simulink model "MultiPointsTrackingWithPhysicalModel_cs"  (Simulink 8.8)
settings: Solver=ode5  StartTime=0.0  StopTime=40  FixedStep=1/20  RelTol=1e-3
model workspace (MAT data in the model file):
  mbox_table.block_array(1).src = 'built-in/Subsystem'
  mbox_table.block_array(1).dest = 'MultiPointsTrackingWithPhysicalModel_cs/Mazda_RX8_1'
  mbox_table.block_array(1).mode = 0
  mbox_table.block_array(2).src = 'simulink/Sinks/Out1'
  mbox_table.block_array(2).dest = 'MultiPointsTrackingWithPhysicalModel_cs/Mazda_RX8_1/STATE_Mazda_RX8_1'
  mbox_table.block_array(2).mode = 0
  mbox_table.block_array(3).src = 'PreScanSimulinkLibrary/State'
  mbox_table.block_array(3).dest = 'MultiPointsTrackingWithPhysicalModel_cs/STATE_Mazda_RX8_1'
  mbox_table.block_array(3).mode = 0
  mbox_table.block_array(4).src = 'PreScanSimulinkLibrary/SELF'
  mbox_table.block_array(4).dest = 'MultiPointsTrackingWithPhysicalModel_cs/SELF_Mazda_RX8_1'
  mbox_table.block_array(4).mode = 0
  mbox_table.block_array(5).src = 'simulink/Sources/In1'
  mbox_table.block_array(5).dest = 'MultiPointsTrackingWithPhysicalModel_cs/Mazda_RX8_1/SELF_Mazda_RX8_1'
  mbox_table.block_array(5).mode = 0
  mbox_table.block_array(6).src = 'PreScanSimulinkLibrary/DemuxSELF'
  mbox_table.block_array(6).dest = 'MultiPointsTrackingWithPhysicalModel_cs/Mazda_RX8_1/SELF_Demux'
  mbox_table.block_array(6).mode = 0
  mbox_table.block_array(7).src = 'built-in/Subsystem'
  mbox_table.block_array(7).dest = 'MultiPointsTrackingWithPhysicalModel_cs/Mazda_RX8_1/Dynamics_Empty'
  mbox_table.block_array(7).mode = 0
  mbox_table.block_array(8).src = 'PreScanSimulinkLibrary/MuxState'
  mbox_table.block_array(8).dest = 'MultiPointsTrackingWithPhysicalModel_cs/Mazda_RX8_1/Dynamics_Empty/MuxState'
  mbox_table.block_array(8).mode = 0
  mbox_table.block_array(9).src = 'simulink/Sinks/Out1'
  mbox_table.block_array(9).dest = 'MultiPointsTrackingWithPhysicalModel_cs/Mazda_RX8_1/Dynamics_Empty/State'
  mbox_table.block_array(9).mode = 0
  mbox_table.block_array(10).src = 'built-in/Note'
  mbox_table.block_array(10).dest = 'MultiPointsTrackingWithPhysicalModel_cs/Mazda_RX8_1/Dynamics_Empty/For state mode ''Dynamic'' positions
    | are not taken into account, as they
    | are computed by integrating velocity.
    | Click annotation for Help.'
  mbox_table.block_array(10).mode = 0
  mbox_table.block_array(11).src = 'SimCoreLibrary/SimCoreConfiguration'
  mbox_table.block_array(11).dest = 'MultiPointsTrackingWithPhysicalModel_cs/SimCoreConfiguration'
  mbox_table.block_array(11).mode = 0
  mbox_table.block_array(12).src = 'SimCoreLibrary/Actuators'
  mbox_table.block_array(12).dest = 'MultiPointsTrackingWithPhysicalModel_cs/Actuators'
  mbox_table.block_array(12).mode = 0
  mbox_table.block_array(13).src = 'SimCoreLibrary/SetActuators'
  mbox_table.block_array(13).dest = 'MultiPointsTrackingWithPhysicalModel_cs/SetActuators'
  mbox_table.block_array(13).mode = 0
  mbox_table.block_array(14).src = 'SimCoreLibrary/GetSensors'
  mbox_table.block_array(14).dest = 'MultiPointsTrackingWithPhysicalModel_cs/GetSensors'
  mbox_table.block_array(14).mode = 0
  mbox_table.block_array(15).src = 'SimCoreLibrary/SimCoreInfo'
  mbox_table.block_array(15).dest = 'MultiPointsTrackingWithPhysicalModel_cs/SimCoreInfo'
  mbox_table.block_array(15).mode = 0
  mbox_table.block_array(16).src = 'PreScanSimulinkLibrary/Regenerate'
  mbox_table.block_array(16).dest = 'MultiPointsTrackingWithPhysicalModel_cs/Regenerate'
  mbox_table.block_array(16).mode = 0
  mbox_table.block_array(17).src = 'PreScanSimulinkLibrary/Record for Replay  '
  mbox_table.block_array(17).dest = 'MultiPointsTrackingWithPhysicalModel_cs/Record for Replay  '
  mbox_table.block_array(17).mode = 0
  mbox_table.block_array(18).src = 'PreScanSimulinkLibrary/Open Useful Blocks'
  mbox_table.block_array(18).dest = 'MultiPointsTrackingWithPhysicalModel_cs/Open Useful Blocks'
  mbox_table.block_array(18).mode = 0
  mbox_table.block_array(19).src = 'PreScanSimulinkLibrary/PreScan Options   '
  mbox_table.block_array(19).dest = 'MultiPointsTrackingWithPhysicalModel_cs/PreScan Options   '
  mbox_table.block_array(19).mode = 0
  mbox_table.block_array(20).src = 'built-in/Note'
  mbox_table.block_array(20).dest = 'MultiPointsTrackingWithPhysicalModel_cs/Version:                  '
  mbox_table.block_array(20).mode = 0
  mbox_table.block_array(21).src = 'built-in/Note'
  mbox_table.block_array(21).dest = 'MultiPointsTrackingWithPhysicalModel_cs/7.5.1'
  mbox_table.block_array(21).mode = 0
  mbox_table.block_array(22).src = 'built-in/Note'
  mbox_table.block_array(22).dest = 'MultiPointsTrackingWithPhysicalModel_cs/Author(s):                '
  mbox_table.block_array(22).mode = 0
  mbox_table.block_array(23).src = 'built-in/Note'
  mbox_table.block_array(23).dest = 'MultiPointsTrackingWithPhysicalModel_cs/N.A.'
  mbox_table.block_array(23).mode = 0
  mbox_table.block_array(24).src = 'built-in/Note'
  mbox_table.block_array(24).dest = 'MultiPointsTrackingWithPhysicalModel_cs/Descriptive text:      '
  mbox_table.block_array(24).mode = 0
  mbox_table.block_array(25).src = 'built-in/Note'
  mbox_table.block_array(25).dest = 'MultiPointsTrackingWithPhysicalModel_cs/N.A.'
  mbox_table.block_array(25).mode = 0
  mbox_table.block_array(26).src = 'built-in/Note'
  mbox_table.block_array(26).dest = 'MultiPointsTrackingWithPhysicalModel_cs/ID
    | 
    | 1'
  mbox_table.block_array(26).mode = 0
  mbox_table.block_array(27).src = 'built-in/Note'
  mbox_table.block_array(27).dest = 'MultiPointsTrackingWithPhysicalModel_cs/OBU-Beacon ID
    | 
    | '
  mbox_table.block_array(27).mode = 0
  mbox_table.block_array(28).src = 'built-in/Note'
  mbox_table.block_array(28).dest = 'MultiPointsTrackingWithPhysicalModel_cs/TypeID
    | 
    | 1'
  mbox_table.block_array(28).mode = 0
  mbox_table.block_array(29).src = 'built-in/Note'
  mbox_table.block_array(29).dest = 'MultiPointsTrackingWithPhysicalModel_cs/TypeTag
    | 
    | Car'
  mbox_table.block_array(29).mode = 0
  mbox_table.block_array(30).src = 'built-in/Note'
  mbox_table.block_array(30).dest = 'MultiPointsTrackingWithPhysicalModel_cs/SD
    | 
    | Y'
  mbox_table.block_array(30).mode = 0
  mbox_table.block_array(31).src = 'built-in/Note'
  mbox_table.block_array(31).dest = 'MultiPointsTrackingWithPhysicalModel_cs/CD
    | 
    | N'
  mbox_table.block_array(31).mode = 0
  mbox_table.block_array(32).src = 'built-in/Note'
  mbox_table.block_array(32).dest = 'MultiPointsTrackingWithPhysicalModel_cs/Name
    | 
    | Mazda_RX8_1'
  mbox_table.block_array(32).mode = 0
  mbox_table.block_array(33).src = 'built-in/Note'
  mbox_table.block_array(33).dest = 'MultiPointsTrackingWithPhysicalModel_cs/Num ID       OBU-Beacon ID     Type ID      Type Tag             SD        CD             Name                          '
  mbox_table.block_array(33).mode = 0
  mbox_table.block_array(34).src = 'built-in/Ground'
  mbox_table.block_array(34).dest = 'MultiPointsTrackingWithPhysicalModel_cs/Mazda_RX8_1/Dynamics_Empty/Ground_1'
  mbox_table.block_array(34).mode = 1
  mbox_table.block_array(35).src = 'built-in/Ground'
  mbox_table.block_array(35).dest = 'MultiPointsTrackingWithPhysicalModel_cs/Mazda_RX8_1/Dynamics_Empty/Ground_2'
  mbox_table.block_array(35).mode = 1
  mbox_table.block_array(36).src = 'built-in/Ground'
  mbox_table.block_array(36).dest = 'MultiPointsTrackingWithPhysicalModel_cs/Mazda_RX8_1/Dynamics_Empty/Ground_3'
  mbox_table.block_array(36).mode = 1
  mbox_table.block_array(37).src = 'built-in/Ground'
  mbox_table.block_array(37).dest = 'MultiPointsTrackingWithPhysicalModel_cs/Mazda_RX8_1/Dynamics_Empty/Ground_4'
  mbox_table.block_array(37).mode = 1
  mbox_table.block_array(38).src = 'built-in/Terminator'
  mbox_table.block_array(38).dest = 'MultiPointsTrackingWithPhysicalModel_cs/Mazda_RX8_1/Terminator_1'
  mbox_table.block_array(38).mode = 1
  mbox_table.block_array(39).src = 'built-in/Terminator'
  mbox_table.block_array(39).dest = 'MultiPointsTrackingWithPhysicalModel_cs/Mazda_RX8_1/Terminator_2'
  mbox_table.block_array(39).mode = 1
  mbox_table.block_array(40).src = 'built-in/Terminator'
  mbox_table.block_array(40).dest = 'MultiPointsTrackingWithPhysicalModel_cs/Mazda_RX8_1/Terminator_3'
  mbox_table.block_array(40).mode = 1
  mbox_table.block_array(41).src = 'built-in/Terminator'
  mbox_table.block_array(41).dest = 'MultiPointsTrackingWithPhysicalModel_cs/Mazda_RX8_1/Terminator_4'
  mbox_table.block_array(41).mode = 1
  mbox_table.block_array(42).src = 'built-in/Terminator'
  mbox_table.block_array(42).dest = 'MultiPointsTrackingWithPhysicalModel_cs/Mazda_RX8_1/Terminator_5'
  mbox_table.block_array(42).mode = 1
  mbox_table.block_array(43).src = 'built-in/Terminator'
  mbox_table.block_array(43).dest = 'MultiPointsTrackingWithPhysicalModel_cs/Mazda_RX8_1/Terminator_6'
  mbox_table.block_array(43).mode = 1
  mbox_table.block_array(44).src = 'built-in/Terminator'
  mbox_table.block_array(44).dest = 'MultiPointsTrackingWithPhysicalModel_cs/Mazda_RX8_1/Terminator_7'
  mbox_table.block_array(44).mode = 1
  mbox_table.block_array(45).src = 'built-in/Terminator'
  mbox_table.block_array(45).dest = 'MultiPointsTrackingWithPhysicalModel_cs/Mazda_RX8_1/Terminator_8'
  mbox_table.block_array(45).mode = 1
  mbox_table.block_index : java.util.Hashtable (value not decoded)
  mbox_table.line_array(1).sys = 'MultiPointsTrackingWithPhysicalModel_cs'
  mbox_table.line_array(1).line_id = 'L1'
  mbox_table.line_array(1).iport = 'STATE_Mazda_RX8_1/1'
  mbox_table.line_array(1).oport = 'Mazda_RX8_1/1'
  mbox_table.line_array(1).mode = 0
  mbox_table.line_array(2).sys = 'MultiPointsTrackingWithPhysicalModel_cs'
  mbox_table.line_array(2).line_id = 'L2'
  mbox_table.line_array(2).iport = 'Mazda_RX8_1/1'
  mbox_table.line_array(2).oport = 'SELF_Mazda_RX8_1/1'
  mbox_table.line_array(2).mode = 0
  mbox_table.line_array(3).sys = 'MultiPointsTrackingWithPhysicalModel_cs/Mazda_RX8_1'
  mbox_table.line_array(3).line_id = 'L3'
  mbox_table.line_array(3).iport = 'SELF_Demux/1'
  mbox_table.line_array(3).oport = 'SELF_Mazda_RX8_1/1'
  mbox_table.line_array(3).mode = 0
  mbox_table.line_array(4).sys = 'MultiPointsTrackingWithPhysicalModel_cs/Mazda_RX8_1/Dynamics_Empty'
  mbox_table.line_array(4).line_id = 'L4'
  mbox_table.line_array(4).iport = 'State/1'
  mbox_table.line_array(4).oport = 'MuxState/1'
  mbox_table.line_array(4).mode = 0
  mbox_table.line_array(5).sys = 'MultiPointsTrackingWithPhysicalModel_cs/Mazda_RX8_1'
  mbox_table.line_array(5).line_id = 'L5'
  mbox_table.line_array(5).iport = 'STATE_Mazda_RX8_1/1'
  mbox_table.line_array(5).oport = 'Dynamics_Empty/1'
  mbox_table.line_array(5).mode = 0
  mbox_table.line_array(6).sys = 'MultiPointsTrackingWithPhysicalModel_cs/Mazda_RX8_1/Dynamics_Empty'
  mbox_table.line_array(6).line_id = 'l1'
  mbox_table.line_array(6).iport = 'MuxState/3'
  mbox_table.line_array(6).oport = 'Ground_1/1'
  mbox_table.line_array(6).mode = 1
  mbox_table.line_array(7).sys = 'MultiPointsTrackingWithPhysicalModel_cs/Mazda_RX8_1/Dynamics_Empty'
  mbox_table.line_array(7).line_id = 'l2'
  mbox_table.line_array(7).iport = 'MuxState/6'
  mbox_table.line_array(7).oport = 'Ground_2/1'
  mbox_table.line_array(7).mode = 1
  mbox_table.line_array(8).sys = 'MultiPointsTrackingWithPhysicalModel_cs/Mazda_RX8_1/Dynamics_Empty'
  mbox_table.line_array(8).line_id = 'l3'
  mbox_table.line_array(8).iport = 'MuxState/7'
  mbox_table.line_array(8).oport = 'Ground_3/1'
  mbox_table.line_array(8).mode = 1
  mbox_table.line_array(9).sys = 'MultiPointsTrackingWithPhysicalModel_cs/Mazda_RX8_1/Dynamics_Empty'
  mbox_table.line_array(9).line_id = 'l4'
  mbox_table.line_array(9).iport = 'MuxState/8'
  mbox_table.line_array(9).oport = 'Ground_4/1'
  mbox_table.line_array(9).mode = 1
  mbox_table.line_array(10).sys = 'MultiPointsTrackingWithPhysicalModel_cs/Mazda_RX8_1'
  mbox_table.line_array(10).line_id = 'l5'
  mbox_table.line_array(10).iport = 'Terminator_1/1'
  mbox_table.line_array(10).oport = 'SELF_Demux/3'
  mbox_table.line_array(10).mode = 1
  mbox_table.line_array(11).sys = 'MultiPointsTrackingWithPhysicalModel_cs/Mazda_RX8_1'
  mbox_table.line_array(11).line_id = 'l6'
  mbox_table.line_array(11).iport = 'Terminator_2/1'
  mbox_table.line_array(11).oport = 'SELF_Demux/4'
  mbox_table.line_array(11).mode = 1
  mbox_table.line_array(12).sys = 'MultiPointsTrackingWithPhysicalModel_cs/Mazda_RX8_1'
  mbox_table.line_array(12).line_id = 'l7'
  mbox_table.line_array(12).iport = 'Terminator_3/1'
  mbox_table.line_array(12).oport = 'SELF_Demux/5'
  mbox_table.line_array(12).mode = 1
  mbox_table.line_array(13).sys = 'MultiPointsTrackingWithPhysicalModel_cs/Mazda_RX8_1'
  mbox_table.line_array(13).line_id = 'l8'
  mbox_table.line_array(13).iport = 'Terminator_4/1'
  mbox_table.line_array(13).oport = 'SELF_Demux/7'
  mbox_table.line_array(13).mode = 1
  mbox_table.line_array(14).sys = 'MultiPointsTrackingWithPhysicalModel_cs/Mazda_RX8_1'
  mbox_table.line_array(14).line_id = 'l9'
  mbox_table.line_array(14).iport = 'Terminator_5/1'
  mbox_table.line_array(14).oport = 'SELF_Demux/8'
  mbox_table.line_array(14).mode = 1
  mbox_table.line_array(15).sys = 'MultiPointsTrackingWithPhysicalModel_cs/Mazda_RX8_1'
  mbox_table.line_array(15).line_id = 'l10'
  mbox_table.line_array(15).iport = 'Terminator_6/1'
  mbox_table.line_array(15).oport = 'SELF_Demux/9'
  mbox_table.line_array(15).mode = 1
  mbox_table.line_array(16).sys = 'MultiPointsTrackingWithPhysicalModel_cs/Mazda_RX8_1'
  mbox_table.line_array(16).line_id = 'l11'
  mbox_table.line_array(16).iport = 'Terminator_7/1'
  mbox_table.line_array(16).oport = 'SELF_Demux/10'
  mbox_table.line_array(16).mode = 1
  mbox_table.line_array(17).sys = 'MultiPointsTrackingWithPhysicalModel_cs/Mazda_RX8_1'
  mbox_table.line_array(17).line_id = 'l12'
  mbox_table.line_array(17).iport = 'Terminator_8/1'
  mbox_table.line_array(17).oport = 'SELF_Demux/12'
  mbox_table.line_array(17).mode = 1
  mbox_table.line_index : java.util.Hashtable (value not decoded)
  mbox_table.next_linenr = 6
  mbox_table.next_termlinenr = 13
  model_closed = 0
  sim_status = 0
PreLoadFcn:
  | check_NUTS_defined;
  | 
  | assignin('base',['model_closed_' bdroot],false);
InitFcn:
  | PreScanExperimentInitFcn(bdroot)
StopFcn:
  | PreScanExperimentStopFcn(bdroot)
undefined symbols (not defined in the file): DiscIntNeverNeededParam, lf, lr
libraries: PreScanSimulinkLibrary x2, PreScanUsefulBlocks x1
CloseFcn:
  | evalin('base',['clear model_closed_' bdroot]);
settings Model: Creator=PRESCAN  LastModifiedBy=yuntao891011
settings OptimizationCC: ExpressionDepthLimit=2147483647  InitFltsAndDblsToZero=on
settings DebuggingCC: SaveWithParameterizedLinksMsg=none  SignalResolutionControl=TryResolveAllWithWarning  MultiTaskDSMMsg=warning  MultiTaskCondExecSysMsg=none
settings GRTTargetCC: TargetFcnLib=ansi_tfl_tmw.mat

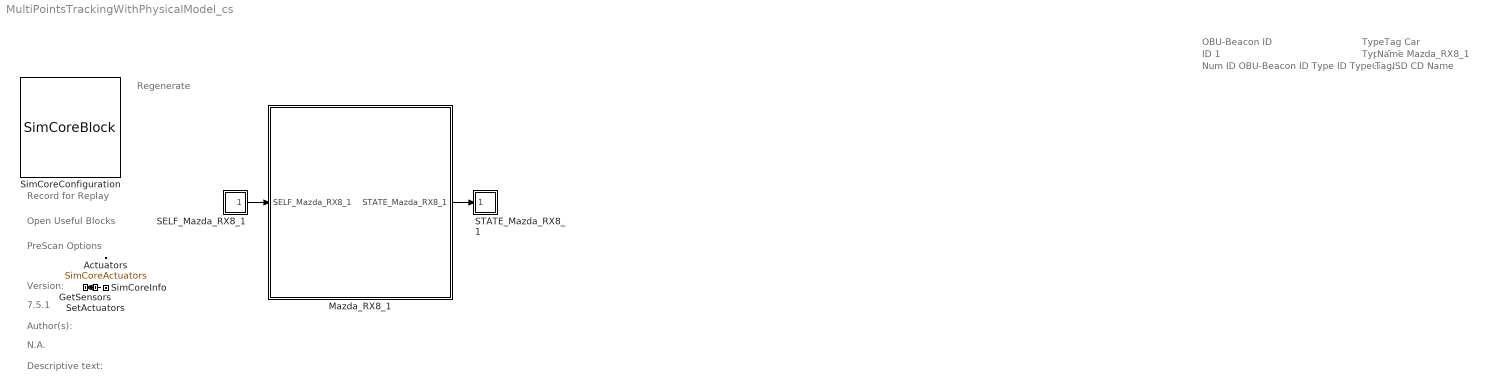
== system MultiPointsTrackingWithPhysicalModel_cs ==
  note: Regenerate
  note: Record for Replay
  note: Open Useful Blocks
  note: PreScan Options
  note: Version:
  note: 7.5.1
  note: Author(s):
  note: N.A.
  note: Descriptive text:
  note: ID
      |
      | 1
  note: OBU-Beacon ID
  note: TypeID
      |
      | 1
  note: TypeTag
      |
      | Car
  note: SD
      |
      | Y
  note: CD
      |
      | N
  note: Name
      |
      | Mazda_RX8_1
  note: Num ID OBU-Beacon ID Type ID Type Tag SD CD Name
  Actuators : DataStoreMemory  DataStoreName=SimCoreActuators  InitialValue=zeros(15,1)  ShowAdditionalParam=off
  GetSensors : Subsystem  Tag=GetSensors  Priority=2  mask(PreScan Simulation Core Block){NrOfSensors=8, TimeStep=1/20}
      mask prompts: NrOfSensors "Number of sensor values"; TimeStep "Timestep [s]"
      mask help:
      | Please do not remove this block from the PreScan compilation sheet,
      | as it contains essential configuration parameters for a PreScan simulation.
      settings: DeleteFcn=PreScanBlockDeleteFcn;
  Mazda_RX8_1 : Subsystem  Tag=WorldObjectSubSystem  InitFcn=UniqueId = '13';
      mask Display: image(imread('Mazda_RX8.jpg'));color('white');text(0,0,' ID=1\n')
  SELF_Mazda_RX8_1 : Subsystem  Tag=SELF  Priority=3  mask(PreScan Source Block: SELF){PortName=SELF_Mazda_RX8_1, PortIndex=0, PortWidth=8, TimeStep=1/20}
      mask prompts: PortName "Auto-Assigned: Port Name [-]"; PortIndex "Auto-Assigned: Port Index [-]"; PortWidth "Auto-Assigned: Port Dimensions"; TimeStep "Auto-Assigned: Upload Period [s]"
      mask help:
      | The SELF port shows (state) information of the actor itself. The outputs are position in the experiment's axis system and the GPS coordinates, and the object's absolute velocity and compass heading.
      |
      | For more information, please click Help.
      settings: DeleteFcn=PreScanBlockDeleteFcn;
      mask Help: eval('openHelp(462)')
      mask Display: image(imread('GPS.png'))
  STATE_Mazda_RX8_1 : Subsystem  Tag=State  Priority=0  mask(PreScan Sink Block: State){x0=34.980075836181641, y0=20.47808837890625, z0=0.51, Roll0=0, Pitch0=0, Yaw0=0, TimeStep=1/20}
      mask prompts: x0 "Ini x-position VEHICLE wrt GLOBAL axis system [m]"; y0 "Ini y-position VEHICLE wrt GLOBAL axis system [m]"; z0 "Ini z-position VEHICLE wrt GLOBAL axis system [m]"; Roll0 "Ini roll-angle BODY wrt VEHICLE axis system [deg]"; Pitch0 "Ini pitch-angle BODY wrt VEHICLE axis system [deg]"; Yaw0 "Ini yaw-angle VEHICLE wrt GLOBAL axis system [deg]"; TimeStep "Time Step [s]"
      mask help:
      | The Actor State contains a vector signal of size (9x1), containing the following signals:
      |
      | -  Position                  (x,y,z)                                     [m]
      | -  Velocity                  (vx,vy,vz)                               [m/s]
      | -  Angles                    (Roll, Pitch, Yaw)                   [rad]
      |
      | The Actor state is defined in the global axis system.
      | The state is superponed on the Initial position defined in the GUI.
      |
      | For more information, please click Help.
      settings: DeleteFcn=PreScanBlockDeleteFcn;
      mask Help: eval('openHelp(222)')
      mask Display: image(imread('State.png'))
  SetActuators : Subsystem  Tag=SetActuators  Priority=1  mask(PreScan Simulation Core Block){TimeStep=1/20, NrOfActuators=15}
      mask prompts: TimeStep "Timestep [s]"; NrOfActuators "Number of actuator values"
      mask help:
      | Please do not remove this block from the PreScan compilation sheet,
      | as it contains essential configuration parameters for a PreScan simulation.
      settings: DeleteFcn=PreScanBlockDeleteFcn;
  SimCoreConfiguration : M-S-Function  Tag=SimCoreConfiguration  Description=C94D2F6BE556C758A06BE63D65435D148AE299C2DC3E9AB8226DE295F427155E  FunctionName=SimCoreBlock  Parameters=ExperimentXML PortsXML SimulationCore HostName CheckStart EnableLog RfR EnableGPUAccel ShowComputationTime  mask(PreScan Simulation Core Configurator){SimulationCore=NUTS, HostName=0, CheckStart=0, prescanversion='7.5.1', EnableLog=off, RfR=0, EnableGPUAccel=off, ShowComputationTime=off}
      mask prompts: SimulationCore "Simulation Core"; HostName "Simulation Host"; CheckStart "Show START Dialog"; prescanversion "PreScan Version"; EnableLog "Create TA Log"; RfR "Record for Replay"; EnableGPUAccel "Enable GPU Acceleration"; ShowComputationTime "Show ComputationTime Scope"
      mask help:
      | Please do not remove this block from the PreScan compilation sheet,
      | as it contains essential configuration parameter for a PreScan simulation.
      mask init:
      | model = bdroot;
      | ExperimentXML = [model(1:end-3) '.pex'];
      | PortsXML = [model '_ports.pcd'];
      settings: DeleteFcn=PreScanBlockDeleteFcn;  ModelCloseFcn=assignin('base',['model_closed_' bdroot],true);
      mask Help: eval('openHelp(812)')
      mask Display: image(imread('prescanlogo.ico'))
  SimCoreInfo : Subsystem  Tag=SimCoreInfo
  wires:
  SetActuators/1(dummy) -> GetSensors/1(dummy)
  Mazda_RX8_1/1(STATE_Mazda_RX8_1) -> STATE_Mazda_RX8_1/1(State)
  SELF_Mazda_RX8_1/1(U) -> Mazda_RX8_1/1(SELF_Mazda_RX8_1)

== system MultiPointsTrackingWithPhysicalModel_cs/GetSensors ==
  dummy : Inport
  GetSensors : M-S-Function  FunctionName=GetSensorsBlock  Parameters=TimeStep NrOfSensors
  tag scope: SimCoreSensors=global
  wires:
  GetSensors/1 -> [SimCoreSensors]
  dummy/1 -> GetSensors/1

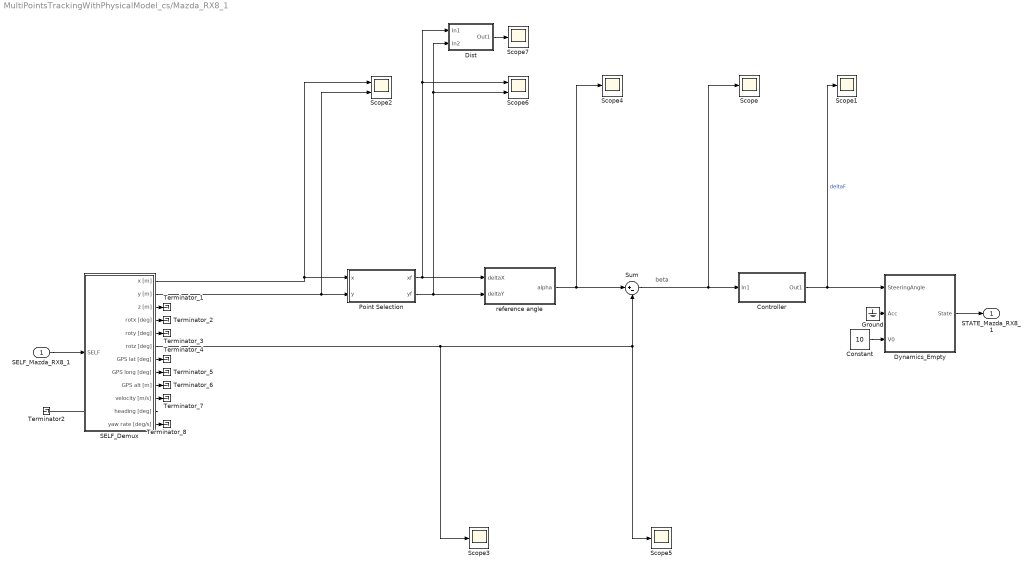
== system MultiPointsTrackingWithPhysicalModel_cs/Mazda_RX8_1 ==
  note: beta
  SELF_Mazda_RX8_1 : Inport  Tag=SELFInport
  Constant : Constant  Value=10
  Controller : Subsystem
  Dist : Subsystem
  Dynamics_Empty : Subsystem  Tag=Dynamics_Empty
      mask Display: port_label('output', 1, 'State');text(0,0,' Empty\n')
  Ground : Ground
  Point Selection : Subsystem
  SELF_Demux : Subsystem  Tag=DemuxSELF  mask(PreScan Demux Block:){}
      settings: DeleteFcn=PreScanBlockDeleteFcn;
      mask Display:
      | port_label('output',1,'x [m]')
      | port_label('output',2,'y [m]')
      | port_label('output',3,'z [m]','texmode','on')
      | port_label('output',4,'Rotx [deg]','texmode','on')
      | port_label('output',5,'Roty [deg]','texmode','on')
      | port_label('output',6,'Rotz [deg]','texmode','on')
      | port_label('output',7,'GPS lat [deg]','texmode','on')
      | port_label('output',8,'GPS long [deg]','texmode','on')
      | port_label('output',9,'GPS alt [m]','texmode','on')
      | port_label('output',10,'Velocity [m/s]')
      | port_label('output',11,'Heading [deg]')
      | port_label('output',12,'Yaw rate [deg/s]')
  Scope{,1,3..5,7} (6 alike) : Scope
  Scope2 : Scope  NumInputPorts=2
  Scope6 : Scope  NumInputPorts=2
  Sum : Sum  Inputs=|+-
  Terminator2 : Terminator
  Terminator_{1..8} (8 alike) : Terminator
  reference angle : Subsystem
  STATE_Mazda_RX8_1 : Outport  Tag=StateOutport
  wires:
  SELF_Demux/1(x [m]) -> Scope2/1, Point Selection/1(x)
  SELF_Demux/2(y [m]) -> Point Selection/2(y), Scope2/2
  Constant/1 -> Dynamics_Empty/3(V0)
  Ground/1 -> Dynamics_Empty/2("Acc ")
  reference angle/1(alpha) -> Sum/1, Scope4/1
  Sum/1 -> Controller/1(In1), Scope/1
  Controller/1(Out1) -> Dynamics_Empty/1(SteeringAngle), Scope1/1  "deltaF"
  SELF_Demux/6(rotz [deg]) -> Scope5/1, Sum/2, Scope3/1
  SELF_Demux/11(heading [deg]) -> Terminator2/1
  Point Selection/1(xf) -> reference angle/1(deltaX), Dist/1(In1), Scope6/1
  Point Selection/2(yf) -> reference angle/2(deltaY), Dist/2(In2), Scope6/2
  Dist/1(Out1) -> Scope7/1
  SELF_Mazda_RX8_1/1 -> SELF_Demux/1(SELF)
  Dynamics_Empty/1(State) -> STATE_Mazda_RX8_1/1
  SELF_Demux/3(z [m]) -> Terminator_1/1
  SELF_Demux/4(rotx [deg]) -> Terminator_2/1
  SELF_Demux/5(roty [deg]) -> Terminator_3/1
  SELF_Demux/7(GPS lat [deg]) -> Terminator_4/1
  SELF_Demux/8(GPS long [deg]) -> Terminator_5/1
  SELF_Demux/9(GPS alt [m]) -> Terminator_6/1
  SELF_Demux/10(velocity [m/s]) -> Terminator_7/1
  SELF_Demux/12(yaw rate [deg/s]) -> Terminator_8/1

== system MultiPointsTrackingWithPhysicalModel_cs/SELF_Mazda_RX8_1 ==
  Selector : Selector  IndexMode=Zero-based  IndexOptions=Starting index (dialog)  Indices=PortIndex  OutputSizes=PortWidth(1)
  U : Outport
  wires:
  Selector/1 -> U/1
  [SimCoreSensors] -> Selector/1

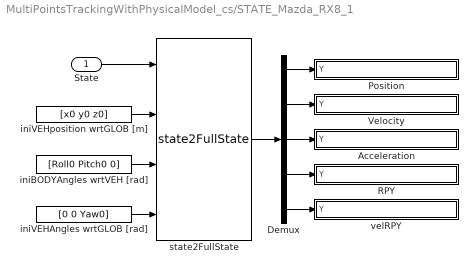
== system MultiPointsTrackingWithPhysicalModel_cs/STATE_Mazda_RX8_1 ==
  State : Inport  SampleTime=TimeStep
  Acceleration : Subsystem  mask(ToSensorWorld){PortName=Acceleration_Mazda_RX8_1, PortIndex=6, PortWidth=3, TimeStep=1/20}
      mask prompts: PortName "Port Name [-]"; PortIndex "Index [-]"; PortWidth "Port Dimensions [-]"; TimeStep "Upload Period [s]"
      mask help: Sends signal(s) from Simulink to the Sensor World
      mask Help:
      | Sends signal(s) from Simulink to the Sensor World.
      | 
      | - Port Name [-]: specifies the name of the output terminal of the Simulink block.
      | - Index [-]: specifies the start position in the output vector sent to the Sensor World
      | - Port dimensions [-]: specifies the width (number of scalars) of the output port
      | - Upload period [s]: specifies the upload period (in seconds) of the port.
      mask Display: port_label('input', 1, PortName)
  Demux : Demux  Outputs=5
  Position : Subsystem  mask(ToSensorWorld){PortName=Position_Mazda_RX8_1, PortIndex=0, PortWidth=3, TimeStep=1/20}
      mask prompts: PortName "Port Name [-]"; PortIndex "Index [-]"; PortWidth "Port Dimensions [-]"; TimeStep "Upload Period [s]"
      mask help: Sends signal(s) from Simulink to the Sensor World
      mask Help:
      | Sends signal(s) from Simulink to the Sensor World.
      | 
      | - Port Name [-]: specifies the name of the output terminal of the Simulink block.
      | - Index [-]: specifies the start position in the output vector sent to the Sensor World
      | - Port dimensions [-]: specifies the width (number of scalars) of the output port
      | - Upload period [s]: specifies the upload period (in seconds) of the port.
      mask Display: port_label('input', 1, PortName)
  RPY : Subsystem  mask(ToSensorWorld){PortName=RPY_Mazda_RX8_1, PortIndex=9, PortWidth=3, TimeStep=1/20}
      mask prompts: PortName "Port Name [-]"; PortIndex "Index [-]"; PortWidth "Port Dimensions [-]"; TimeStep "Upload Period [s]"
      mask help: Sends signal(s) from Simulink to the Sensor World
      mask Help:
      | Sends signal(s) from Simulink to the Sensor World.
      | 
      | - Port Name [-]: specifies the name of the output terminal of the Simulink block.
      | - Index [-]: specifies the start position in the output vector sent to the Sensor World
      | - Port dimensions [-]: specifies the width (number of scalars) of the output port
      | - Upload period [s]: specifies the upload period (in seconds) of the port.
      mask Display: port_label('input', 1, PortName)
  Velocity : Subsystem  mask(ToSensorWorld){PortName=Velocity_Mazda_RX8_1, PortIndex=3, PortWidth=3, TimeStep=1/20}
      mask prompts: PortName "Port Name [-]"; PortIndex "Index [-]"; PortWidth "Port Dimensions [-]"; TimeStep "Upload Period [s]"
      mask help: Sends signal(s) from Simulink to the Sensor World
      mask Help:
      | Sends signal(s) from Simulink to the Sensor World.
      | 
      | - Port Name [-]: specifies the name of the output terminal of the Simulink block.
      | - Index [-]: specifies the start position in the output vector sent to the Sensor World
      | - Port dimensions [-]: specifies the width (number of scalars) of the output port
      | - Upload period [s]: specifies the upload period (in seconds) of the port.
      mask Display: port_label('input', 1, PortName)
  iniBODYAngles wrtVEH [rad] : Constant  Value=[Roll0 Pitch0 0]  SampleTime=TimeStep
  iniVEHAngles wrtGLOB [rad] : Constant  Value=[0 0 Yaw0]  SampleTime=TimeStep
  iniVEHposition wrtGLOB [m] : Constant  Value=[x0 y0 z0]  SampleTime=TimeStep
  state2FullState : PreScanSimulinkLibrary/state2FullState  SystemSampleTime=-1
  velRPY : Subsystem  mask(ToSensorWorld){PortName=velRPY_Mazda_RX8_1, PortIndex=12, PortWidth=3, TimeStep=1/20}
      mask prompts: PortName "Port Name [-]"; PortIndex "Index [-]"; PortWidth "Port Dimensions [-]"; TimeStep "Upload Period [s]"
      mask help: Sends signal(s) from Simulink to the Sensor World
      mask Help:
      | Sends signal(s) from Simulink to the Sensor World.
      | 
      | - Port Name [-]: specifies the name of the output terminal of the Simulink block.
      | - Index [-]: specifies the start position in the output vector sent to the Sensor World
      | - Port dimensions [-]: specifies the width (number of scalars) of the output port
      | - Upload period [s]: specifies the upload period (in seconds) of the port.
      mask Display: port_label('input', 1, PortName)
  wires:
  Demux/5 -> velRPY/1(Y)
  Demux/4 -> RPY/1(Y)
  Demux/3 -> Acceleration/1(Y)
  Demux/2 -> Velocity/1(Y)
  Demux/1 -> Position/1(Y)
  State/1 -> state2FullState/1
  state2FullState/1 -> Demux/1
  iniVEHposition wrtGLOB [m]/1 -> state2FullState/2
  iniBODYAngles wrtVEH [rad]/1 -> state2FullState/3
  iniVEHAngles wrtGLOB [rad]/1 -> state2FullState/4

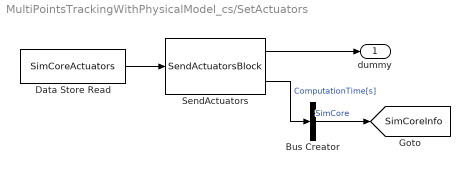
== system MultiPointsTrackingWithPhysicalModel_cs/SetActuators ==
  Bus Creator : BusCreator  Inputs=1
  Data Store Read : DataStoreRead  DataStoreName=SimCoreActuators  SampleTime=TimeStep
  SendActuators : M-S-Function  FunctionName=SendActuatorsBlock  Parameters=TimeStep NrOfActuators
  dummy : Outport
  tag scope: SimCoreInfo=global
  wires:
  Bus Creator/1 -> [SimCoreInfo]  "SimCore"
  SendActuators/2 -> Bus Creator/1  "ComputationTime[s]"
  SendActuators/1 -> dummy/1
  Data Store Read/1 -> SendActuators/1

== system MultiPointsTrackingWithPhysicalModel_cs/SimCoreInfo ==
  Bus Selector : BusSelector  OutputSignals=ComputationTime[s]
  Time : Scope
  wires:
  Bus Selector/1 -> Time/1  "<ComputationTime[s]>"
  [SimCoreInfo] -> Bus Selector/1

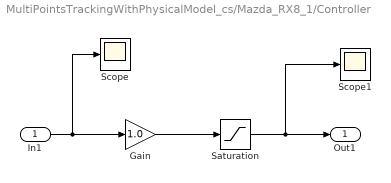
== system MultiPointsTrackingWithPhysicalModel_cs/Mazda_RX8_1/Controller ==
  In1 : Inport
  Gain : Gain  Gain=1.0
  Saturation : Saturate  UpperLimit=90  LowerLimit=-90
  Scope : Scope
  Scope1 : Scope
  Out1 : Outport
  wires:
  In1/1 -> Gain/1, Scope/1
  Saturation/1 -> Scope1/1, Out1/1
  Gain/1 -> Saturation/1

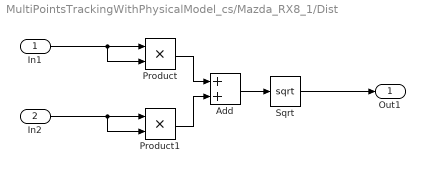
== system MultiPointsTrackingWithPhysicalModel_cs/Mazda_RX8_1/Dist ==
  In1 : Inport
  In2 : Inport  Port=2
  Add : Sum
  Product : Product
  Product1 : Product
  Sqrt : Sqrt  SaturateOnIntegerOverflow=on
  Out1 : Outport
  wires:
  In1/1 -> Product/2, Product/1
  In2/1 -> Product1/2, Product1/1
  Product/1 -> Add/1
  Product1/1 -> Add/2
  Sqrt/1 -> Out1/1
  Add/1 -> Sqrt/1

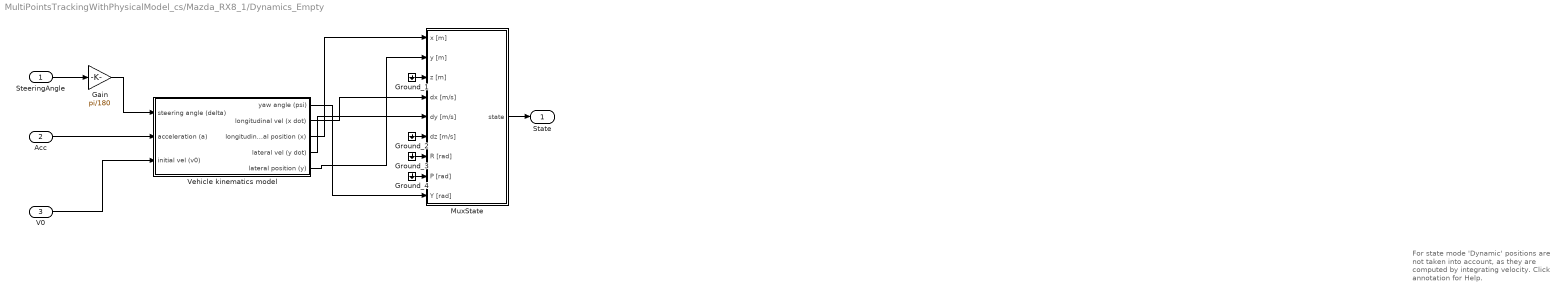
== system MultiPointsTrackingWithPhysicalModel_cs/Mazda_RX8_1/Dynamics_Empty ==
  note: For state mode 'Dynamic' positions
      | are not taken into account, as they
      | are computed by integrating velocity.
      | Click annotation for Help.
  SteeringAngle : Inport
  "Acc " : Inport  Port=2
  V0 : Inport  Port=3
  Gain : Gain  Gain=pi/180
  Ground_{1..4} (4 alike) : Ground
  MuxState : Subsystem  Tag=MuxState  mask(Empty Dynamics State Block){positioningmode=on, TimeStep=1/20}
      mask prompts: positioningmode "Positioning Mode"; TimeStep "Auto Assigned: Time Step [s]"
      mask help:
      | Build the state of an actor based on user input.
      | The user can either use positioning mode or dynamics mode.
      | - When using positioning mode the position and orientation of the actor are set directly based on the input. Expected input is relative to the initial position and orientation of the actor. It's also possible to specify the velocity of the actor, though this input isn't used, only passed on.
      | - When using dynamics mode the position input is ignored. Expected input is velocity and orientation. The velocity is relative the current orientation of the actor, while orientation is relative to its initial orientation. The position of the actor is calculated based on the velocity and orientation given.
      settings: DeleteFcn=PreScanBlockDeleteFcn;
  Vehicle kinematics model : Subsystem
  State : Outport  Tag=StateOutport
  wires:
  Vehicle kinematics model/1(yaw angle (psi)) -> MuxState/9(Y [rad])
  Vehicle kinematics model/4(lateral vel (y dot)) -> MuxState/5(dy [m/s])
  "Acc "/1 -> Vehicle kinematics model/2(acceleration (a))
  Vehicle kinematics model/2(longitudinal vel (x dot)) -> MuxState/4(dx [m/s])
  Vehicle kinematics model/3(longitudinal position (x)) -> MuxState/1(x [m])
  V0/1 -> Vehicle kinematics model/3(initial vel (v0))
  Vehicle kinematics model/5(lateral position (y)) -> MuxState/2(y [m])
  Gain/1 -> Vehicle kinematics model/1(steering angle (delta))
  SteeringAngle/1 -> Gain/1
  MuxState/1(state) -> State/1
  Ground_1/1 -> MuxState/3(z [m])
  Ground_2/1 -> MuxState/6(dz [m/s])
  Ground_3/1 -> MuxState/7(R [rad])
  Ground_4/1 -> MuxState/8(P [rad])

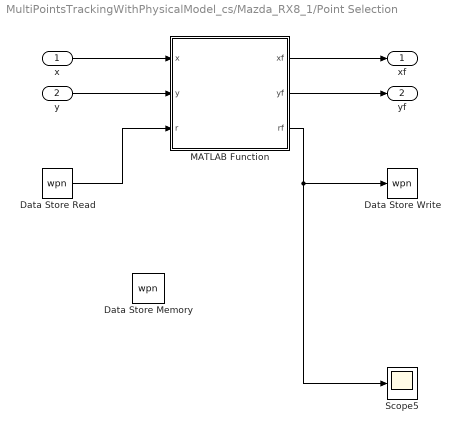
== system MultiPointsTrackingWithPhysicalModel_cs/Mazda_RX8_1/Point Selection ==
  x : Inport
  y : Inport  Port=2
  Data Store Memory : DataStoreMemory  DataStoreName=wpn  ReadBeforeWriteMsg=warning  WriteAfterWriteMsg=warning  WriteAfterReadMsg=warning  InitialValue=1  ShowAdditionalParam=off  OutMin=1  OutMax=10  OutDataTypeStr=double
  Data Store Read : DataStoreRead  DataStoreName=wpn
  Data Store Write : DataStoreWrite  DataStoreName=wpn
  MATLAB Function : MATLAB Function  TreatAsAtomicUnit=on
  Scope5 : Scope
  xf : Outport
  yf : Outport  Port=2
  wires:
  x/1 -> MATLAB Function/1(x)
  y/1 -> MATLAB Function/2(y)
  MATLAB Function/1(xf) -> xf/1
  MATLAB Function/2(yf) -> yf/1
  Data Store Read/1 -> MATLAB Function/3(r)
  MATLAB Function/3(rf) -> Scope5/1, Data Store Write/1

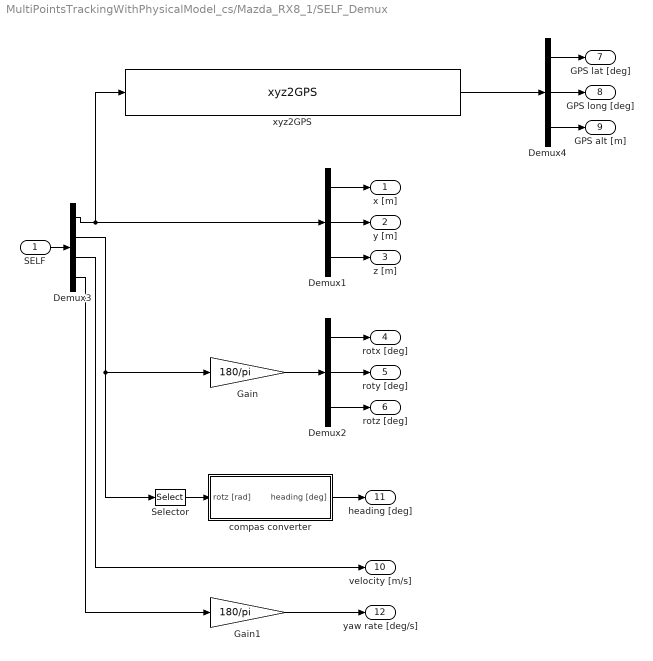
== system MultiPointsTrackingWithPhysicalModel_cs/Mazda_RX8_1/SELF_Demux ==
  SELF : Inport
  Demux1 : Demux  Outputs=3
  Demux2 : Demux  Outputs=3
  Demux3 : Demux  Outputs=[3 3 1 1]
  Demux4 : Demux  Outputs=3
  Gain : Gain  Gain=180/pi
  Gain1 : Gain  Gain=180/pi
  Selector : Selector  InputPortWidth=3  IndexOptions=Index vector (dialog)  Indices=[3]  OutputSizes=1
  compas converter : Subsystem
  xyz2GPS : PreScanUsefulBlocks/xyz2GPS  CoordinateCount=1  GPS_base=[0.000000 0.000000 0.000]
  x [m] : Outport
  y [m] : Outport  Port=2
  z [m] : Outport  Port=3
  rotx [deg] : Outport  Port=4
  roty [deg] : Outport  Port=5
  rotz [deg] : Outport  Port=6
  GPS lat [deg] : Outport  Port=7
  GPS long [deg] : Outport  Port=8
  GPS alt [m] : Outport  Port=9
  velocity [m/s] : Outport  Port=10
  heading [deg] : Outport  Port=11
  yaw rate [deg/s] : Outport  Port=12
  wires:
  Demux3/4 -> Gain1/1
  Gain1/1 -> yaw rate [deg/s]/1
  Demux3/3 -> velocity [m/s]/1
  compas converter/1(heading [deg]) -> heading [deg]/1
  xyz2GPS/1 -> Demux4/1
  Demux4/3 -> GPS alt [m]/1
  Demux4/2 -> GPS long [deg]/1
  Demux4/1 -> GPS lat [deg]/1
  Demux3/2 -> Gain/1, Selector/1
  Demux3/1 -> xyz2GPS/1, Demux1/1
  SELF/1 -> Demux3/1
  Demux2/3 -> rotz [deg]/1
  Demux2/2 -> roty [deg]/1
  Demux2/1 -> rotx [deg]/1
  Demux1/3 -> z [m]/1
  Demux1/2 -> y [m]/1
  Demux1/1 -> x [m]/1
  Gain/1 -> Demux2/1
  Selector/1 -> compas converter/1(rotz [rad])

== system MultiPointsTrackingWithPhysicalModel_cs/Mazda_RX8_1/reference angle ==
  deltaX : Inport
  deltaY : Inport  Port=2
  Trigonometric Function : Trigonometry  Operator=atan2
  rad-degree : Gain  Gain=180/pi
  alpha : Outport
  wires:
  deltaY/1 -> Trigonometric Function/1
  deltaX/1 -> Trigonometric Function/2
  rad-degree/1 -> alpha/1
  Trigonometric Function/1 -> rad-degree/1

== system MultiPointsTrackingWithPhysicalModel_cs/STATE_Mazda_RX8_1/Acceleration ==
  Y : Inport
  Assignment : Assignment  IndexMode=Zero-based  SampleTime=TimeStep  IndexOptions=Starting index (dialog)  Indices=PortIndex  OutputSizes=[1 1]
  Data Store Read : DataStoreRead  DataStoreName=SimCoreActuators  SampleTime=TimeStep
  Data Store Write : DataStoreWrite  DataStoreName=SimCoreActuators
  wires:
  Assignment/1 -> Data Store Write/1
  Data Store Read/1 -> Assignment/1
  Y/1 -> Assignment/2

== system MultiPointsTrackingWithPhysicalModel_cs/STATE_Mazda_RX8_1/Position ==
  Y : Inport
  Assignment : Assignment  IndexMode=Zero-based  SampleTime=TimeStep  IndexOptions=Starting index (dialog)  Indices=PortIndex  OutputSizes=[1 1]
  Data Store Read : DataStoreRead  DataStoreName=SimCoreActuators  SampleTime=TimeStep
  Data Store Write : DataStoreWrite  DataStoreName=SimCoreActuators
  wires:
  Y/1 -> Assignment/2
  Data Store Read/1 -> Assignment/1
  Assignment/1 -> Data Store Write/1

== system MultiPointsTrackingWithPhysicalModel_cs/STATE_Mazda_RX8_1/RPY ==
  Y : Inport
  Assignment : Assignment  IndexMode=Zero-based  SampleTime=TimeStep  IndexOptions=Starting index (dialog)  Indices=PortIndex  OutputSizes=[1 1]
  Data Store Read : DataStoreRead  DataStoreName=SimCoreActuators  SampleTime=TimeStep
  Data Store Write : DataStoreWrite  DataStoreName=SimCoreActuators
  wires:
  Assignment/1 -> Data Store Write/1
  Data Store Read/1 -> Assignment/1
  Y/1 -> Assignment/2

== system MultiPointsTrackingWithPhysicalModel_cs/STATE_Mazda_RX8_1/Velocity ==
  Y : Inport
  Assignment : Assignment  IndexMode=Zero-based  SampleTime=TimeStep  IndexOptions=Starting index (dialog)  Indices=PortIndex  OutputSizes=[1 1]
  Data Store Read : DataStoreRead  DataStoreName=SimCoreActuators  SampleTime=TimeStep
  Data Store Write : DataStoreWrite  DataStoreName=SimCoreActuators
  wires:
  Assignment/1 -> Data Store Write/1
  Data Store Read/1 -> Assignment/1
  Y/1 -> Assignment/2

== system MultiPointsTrackingWithPhysicalModel_cs/STATE_Mazda_RX8_1/velRPY ==
  Y : Inport
  Assignment : Assignment  IndexMode=Zero-based  SampleTime=TimeStep  IndexOptions=Starting index (dialog)  Indices=PortIndex  OutputSizes=[1 1]
  Data Store Read : DataStoreRead  DataStoreName=SimCoreActuators  SampleTime=TimeStep
  Data Store Write : DataStoreWrite  DataStoreName=SimCoreActuators
  wires:
  Assignment/1 -> Data Store Write/1
  Data Store Read/1 -> Assignment/1
  Y/1 -> Assignment/2

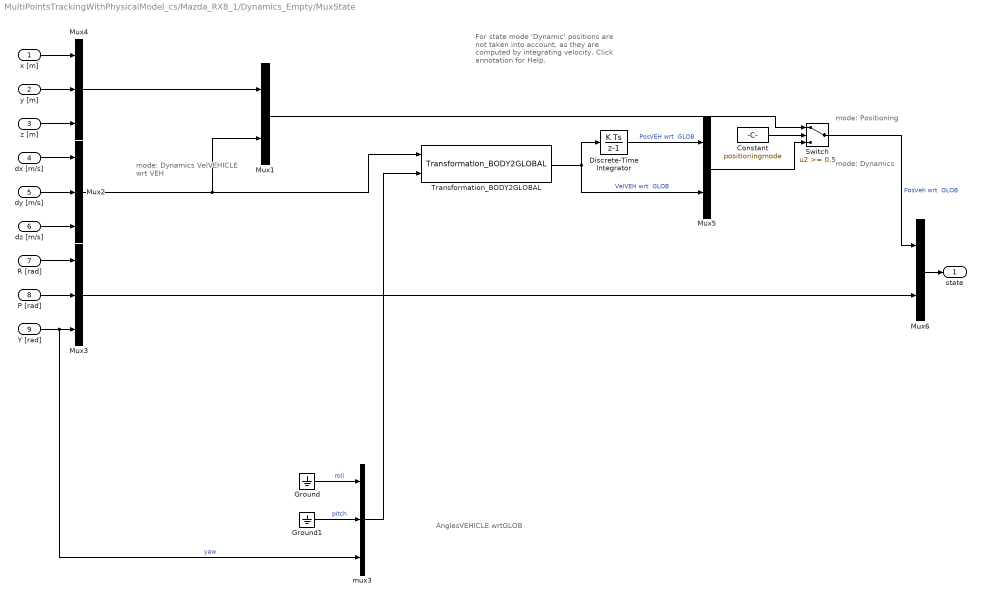
== system MultiPointsTrackingWithPhysicalModel_cs/Mazda_RX8_1/Dynamics_Empty/MuxState ==
  note: mode: Dynamics
  note: mode: Positioning
  note: mode: Dynamics
      | VelVEHICLE
      | wrt VEH
  note: AnglesVEHICLE
      | wrtGLOB
  note: For state mode 'Dynamic' positions
      | are not taken into account, as they
      | are computed by integrating velocity.
      | Click annotation for Help.
  x [m] : Inport  SampleTime=TimeStep
  y [m] : Inport  Port=2  SampleTime=TimeStep
  z [m] : Inport  Port=3  SampleTime=TimeStep
  dx [m/s] : Inport  Port=4  SampleTime=TimeStep
  dy [m/s] : Inport  Port=5  SampleTime=TimeStep
  dz [m/s] : Inport  Port=6  SampleTime=TimeStep
  R [rad] : Inport  Port=7  SampleTime=TimeStep
  P [rad] : Inport  Port=8  SampleTime=TimeStep
  Y [rad] : Inport  Port=9  SampleTime=TimeStep
  Constant : Constant  DisableCoverage=on  Value=positioningmode
  Discrete-Time Integrator : DiscreteIntegrator  SampleTime=TimeStep  ICPrevOutput=DiscIntNeverNeededParam  ICPrevScaledInput=DiscIntNeverNeededParam
  Ground : Ground
  Ground1 : Ground
  Mux1 : Mux  Inputs=[3 3]
  Mux2 : Mux  Inputs=3
  Mux3 : Mux  Inputs=3
  Mux4 : Mux  Inputs=3
  Mux5 : Mux  Inputs=[3 3]
  Mux6 : Mux  Inputs=[6 3]
  Switch : Switch  Threshold=0.5
  Transformation_BODY2GLOBAL : PreScanSimulinkLibrary/Simple_Vehicle_Dynamics/Chassis/MuxDynState/Transformation_BODY2GLOBAL
  mux3 : Mux  Inputs=3
  state : Outport
  wires:
  Constant/1 -> Switch/2
  Mux6/1 -> state/1
  Mux4/1 -> Mux1/1
  Mux5/1 -> Switch/3
  Mux1/1 -> Switch/1
  Switch/1 -> Mux6/1  "PosVeh wrt  GLOB"
  P [rad]/1 -> Mux3/2
  R [rad]/1 -> Mux3/1
  dz [m/s]/1 -> Mux2/3
  dy [m/s]/1 -> Mux2/2
  dx [m/s]/1 -> Mux2/1
  z [m]/1 -> Mux4/3
  y [m]/1 -> Mux4/2
  x [m]/1 -> Mux4/1
  Ground1/1 -> mux3/2  "pitch"
  Y [rad]/1 -> mux3/3, Mux3/3  "yaw"
  Mux3/1 -> Mux6/2
  Transformation_BODY2GLOBAL/1 -> Discrete-Time Integrator/1, Mux5/2  "VelVEH wrt  GLOB"
  mux3/1 -> Transformation_BODY2GLOBAL/2
  Ground/1 -> mux3/1  "roll"
  Mux2/1 -> Mux1/2, Transformation_BODY2GLOBAL/1
  Discrete-Time Integrator/1 -> Mux5/1  "PosVEH wrt  GLOB"

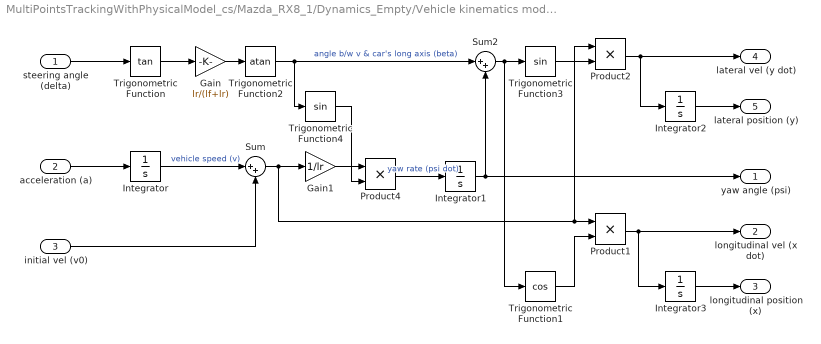
== system MultiPointsTrackingWithPhysicalModel_cs/Mazda_RX8_1/Dynamics_Empty/Vehicle kinematics model ==
  steering angle (delta) : Inport
  acceleration (a) : Inport  Port=2
  initial vel (v0) : Inport  Port=3
  Gain : Gain  Gain=lr/(lf+lr)
  Gain1 : Gain  Gain=1/lr
  Integrator{,1..3} (4 alike) : Integrator
  Product1 : Product
  Product2 : Product
  Product4 : Product
  Sum : Sum  Inputs=|++
  Sum2 : Sum  Inputs=|++
  Trigonometric Function : Trigonometry  Operator=tan
  Trigonometric Function1 : Trigonometry  Operator=cos
  Trigonometric Function2 : Trigonometry  Operator=atan
  Trigonometric Function3 : Trigonometry
  Trigonometric Function4 : Trigonometry
  yaw angle (psi) : Outport
  longitudinal vel (x dot) : Outport  Port=2
  longitudinal position (x) : Outport  Port=3
  lateral vel (y dot) : Outport  Port=4
  lateral position (y) : Outport  Port=5
  wires:
  acceleration (a)/1 -> Integrator/1
  steering angle (delta)/1 -> Trigonometric Function/1
  Trigonometric Function/1 -> Gain/1
  Gain/1 -> Trigonometric Function2/1
  Trigonometric Function2/1 -> Sum2/1, Trigonometric Function4/1  "angle b/w v & car's long axis (beta)"
  Gain1/1 -> Product4/1
  Product4/1 -> Integrator1/1  "yaw rate (psi dot)"
  Sum2/1 -> Trigonometric Function3/1, Trigonometric Function1/1
  Trigonometric Function1/1 -> Product1/2
  Product1/1 -> Integrator3/1, longitudinal vel (x dot)/1
  Trigonometric Function3/1 -> Product2/2
  Product2/1 -> Integrator2/1, lateral vel (y dot)/1
  Integrator2/1 -> lateral position (y)/1
  Integrator3/1 -> longitudinal position (x)/1
  Trigonometric Function4/1 -> Product4/2
  Integrator1/1 -> yaw angle (psi)/1, Sum2/2
  initial vel (v0)/1 -> Sum/2
  Sum/1 -> Product2/1, Product1/1, Gain1/1
  Integrator/1 -> Sum/1  "vehicle speed (v)"

== system MultiPointsTrackingWithPhysicalModel_cs/Mazda_RX8_1/SELF_Demux/compas converter ==
  rotz [rad] : Inport
  cart2compas : Subsystem
  rad2deg : Gain  Gain=180/pi
  heading [deg] : Outport
  wires:
  cart2compas/1(heading [deg]) -> heading [deg]/1
  rotz [rad]/1 -> rad2deg/1
  rad2deg/1 -> cart2compas/1(Angle [deg])

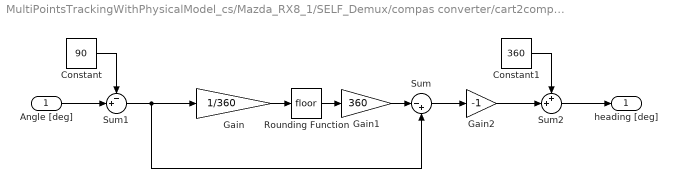
== system MultiPointsTrackingWithPhysicalModel_cs/Mazda_RX8_1/SELF_Demux/compas converter/cart2compas ==
  Angle [deg] : Inport
  Constant : Constant  Value=90
  Constant1 : Constant  Value=360
  Gain : Gain  Gain=1/360
  Gain1 : Gain  Gain=360
  Gain2 : Gain  Gain=-1
  Rounding Function : Rounding
  Sum : Sum  Inputs=|-+
  Sum1 : Sum  Inputs=-+|
  Sum2 : Sum  Inputs=++|
  heading [deg] : Outport
  wires:
  Sum2/1 -> heading [deg]/1
  Constant1/1 -> Sum2/1
  Gain2/1 -> Sum2/2
  Constant/1 -> Sum1/1
  Sum1/1 -> Sum/2, Gain/1
  Sum/1 -> Gain2/1
  Angle [deg]/1 -> Sum1/2
  Gain1/1 -> Sum/1
  Rounding Function/1 -> Gain1/1
  Gain/1 -> Rounding Function/1

== matlab function Mazda_RX8_1/Point Selection/MATLAB Function ==
  data: x input double; xf output double; y input double; yf output double; r input double; rf output double
function [xf,yf,rf] = fcn(x,y,r)

n  = 5;
points = [10 40; 25, 77 ; 84, 60;50 55;-3 -4];
Tolerance=0.5;

xf = 0;
yf = 0;
i = r;

while i <= n
    dist = sqrt((x-points(i,1))^2 + (y-points(i,2))^2);
    if dist<Tolerance
        if i<n
            i=i+1;
        else
            i=1;
        end
    else
        xf = points(i,1)-x;
        yf = points(i,2)-y;     
        break;
    end
    

end

rf = i;

end
